simulink subsystem "LowLevelController"  (R2025a)
settings: Solver=VariableStepAuto  StartTime=0.0  StopTime=10.0  RelTol=1e-3
model mask{motor_km=0}
settings Model: Creator=Глеб  LastModifiedBy=Глеб

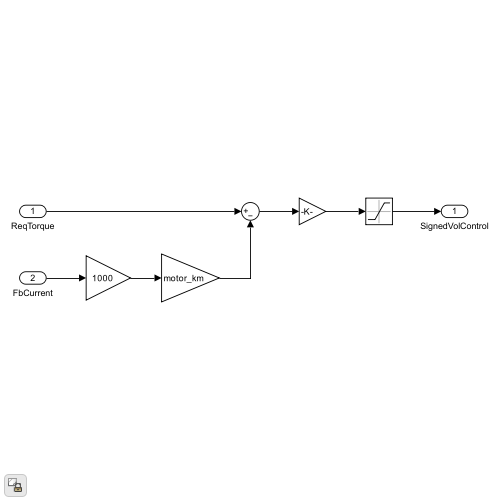
[thumbnail: Simulink's stored preview of the top-level diagram]
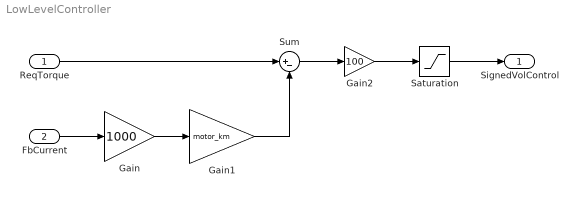
== system LowLevelController ==
  ReqTorque : Inport
  FbCurrent : Inport  Port=2
  Gain : Gain  Gain=1000
  Gain1 : Gain  Gain=motor_km
  Gain2 : Gain  Gain=100
  Saturation : Saturate  UpperLimit=3.3  LowerLimit=-3.3
  Sum : Sum  Inputs=|+-
  SignedVolControl : Outport
  wires:
  Gain1/1 -> Sum/2
  Gain2/1 -> Saturation/1
  Sum/1 -> Gain2/1
  Gain/1 -> Gain1/1
  ReqTorque/1 -> Sum/1
  FbCurrent/1 -> Gain/1
  Saturation/1 -> SignedVolControl/1
